simulink model "Circuit_Diagram"  (R2022a)
settings: Solver=VariableStepAuto  StartTime=0.0  StopTime=10.0  RelTol=1e-3
libraries: fl_lib x27, ee_lib x9
settings Model: Creator=Tony  LastModifiedBy=Tony

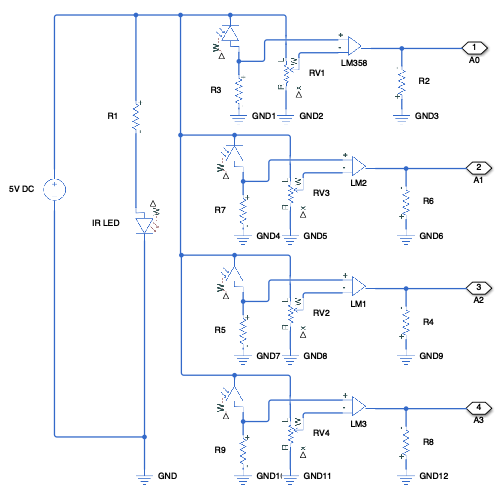
[thumbnail: Simulink's stored preview of the top-level diagram]
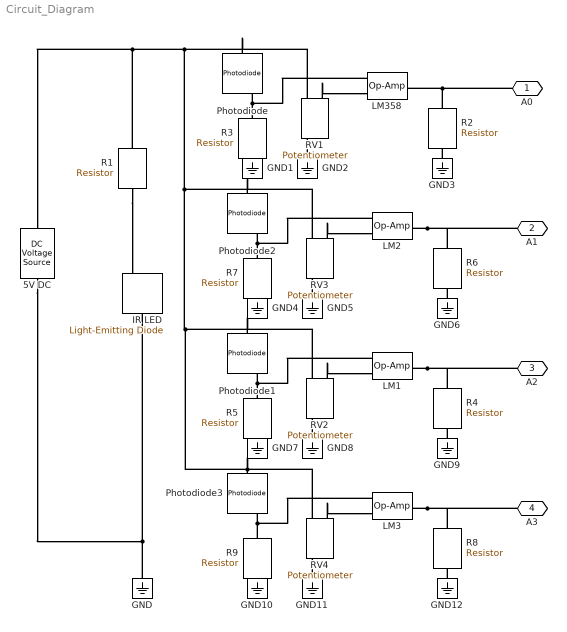
== system Circuit_Diagram ==
  5V DC : fl_lib/Electrical/Electrical Sources/DC Voltage Source  v0=5 V
      settings: SourceProductBaseCode=PW,SS,VE
  GND{,1..12} (13 alike) : fl_lib/Electrical/Electrical Elements/Electrical Reference
      settings: SourceProductBaseCode=PW,SS,VE
  "IR LED " : ee_lib/Sensors & Transducers/Light-Emitting Diode  Gain=0.005 W/A  prmExp=1  I12=[.0017, .003] A  V12=[.9, 1.05] V  IS=5e-5 A  ec=10  RS=0.1 Ohm  Tmeas=25 degC  C_param=1  CJ=20 pF  CJ0=20 pF  VJ=1 V  Mgrad=0.5  Vvec=[.1, 10, 100] V  Cvec=[15, 10, 2] pF  FC=0.5  T_param=1  IS_T2=1.8e-4 A  I1_T2=0.0034 A  V1_T2=1.05 V  Tmeas2=125 degC  EG_param=1  EG=1.11 eV  XTI_param=1  XTI=3  Tdevice=25 degC  i_capacitor_specify=off  i_capacitor_priority=High  i_capacitor=0 A  i_capacitor_nominal_specify=off  i_capacitor_nominal_unit=A  i_capacitor_nominal_value=1  v_capacitor_specify=off  v_capacitor_priority=None  v_capacitor=0 V  v_capacitor_nominal_specify=off  v_capacitor_nominal_unit=V  v_capacitor_nominal_value=1  thermal_network_parameterization=ee.enum.thermalNetworkTopology.junctionCase  Rth=[0, 10] K/W  Rth_Cauer=[1, 3, 10] K/W  Rth_Foster=[4, 6] K/W  thermal_mass_parameterization=ee.enum.thermalNetwork.timeconstant  thermal_mass=[0, 1] J/K  thermal_mass_Cauer=[1.5, 2, 3] J/K  thermal_mass_Foster=[1.5, 3] J/K  thermal_time_constant=[0, 10] s  thermal_time_constant_Cauer=[1, 3, 10] s  thermal_time_constant_Foster=[6, 18] s  thermal_mass_initial_temperatures=[25, 25] degC  thermal_mass_initial_temperatures_Cauer=[25, 25, 25] degC  steadyState_Foster=simscape.enum.onoff.on  Tvec_initial_Foster=[25, 25, 25, 25] degC
      settings: SourceProductBaseCode=PS  InternalSimscapePortConfiguration="{\"Bottom\":[],\"Left\":[{\"id\":\"W\",\"label\":\"W\",\"type\":\"output\"},{\"id\":\"p\",\"label\":\"\",\"type\":\"foundation.electrical.electrical\"}],\"Right\":[{\"id\":\"n\",\"label\":\"\",\"type\":\"foundation.electrical.electrical\"}],\"Top\":[]}"
  LM{1..3,358} (4 alike) : fl_lib/Electrical/Electrical Elements/Op-Amp  outI_specify=off  outI_priority=None  outI=0 A  outI_nominal_specify=off  outI_nominal_unit=A  outI_nominal_value=1
      settings: SourceProductBaseCode=PW,SS,VE
  Photodiode{,1..3} (4 alike) : ee_lib/Sensors & Transducers/Photodiode  prmFlux=1  Imeas=25 uA  FluxD=5 W/m^2  G=5e-6 A*m^2/W  prmExp=1  I2=0.1 A  V2=1.3 V  IS=5e-9 A  ec=3  RS=0.1 Ohm  Tmeas=25 degC  C_param=1  CJ=60 pF  CJ0=60 pF  VJ=1 V  Mgrad=0.5  Vvec=[.1, 10, 100] V  Cvec=[45, 3, 6] pF  FC=0.5  T_param=1  IS_T2=2.5e-7 A  I1_T2=0.07 A  V1_T2=1.3 V  Tmeas2=125 degC  EG_param=1  EG=1.11 eV  XTI_param=1  XTI=3  Tdevice=25 degC  i_capacitor_specify=off  i_capacitor_priority=High  i_capacitor=0 A  i_capacitor_nominal_specify=off  i_capacitor_nominal_unit=A  i_capacitor_nominal_value=1  v_capacitor_specify=off  v_capacitor_priority=None  v_capacitor=0 V  v_capacitor_nominal_specify=off  v_capacitor_nominal_unit=V  v_capacitor_nominal_value=1  thermal_network_parameterization=ee.enum.thermalNetworkTopology.junctionCase  Rth=[0, 10] K/W  Rth_Cauer=[1, 3, 10] K/W  Rth_Foster=[4, 6] K/W  thermal_mass_parameterization=ee.enum.thermalNetwork.timeconstant  thermal_mass=[0, 1] J/K  thermal_mass_Cauer=[1.5, 2, 3] J/K  thermal_mass_Foster=[1.5, 3] J/K  thermal_time_constant=[0, 10] s  thermal_time_constant_Cauer=[1, 3, 10] s  thermal_time_constant_Foster=[6, 18] s  thermal_mass_initial_temperatures=[25, 25] degC  thermal_mass_initial_temperatures_Cauer=[25, 25, 25] degC  steadyState_Foster=simscape.enum.onoff.on  Tvec_initial_Foster=[25, 25, 25, 25] degC
      settings: SourceProductBaseCode=PS  InternalSimscapePortConfiguration="{\"Bottom\":[],\"Left\":[{\"id\":\"W\",\"label\":\"W\",\"type\":\"input\"},{\"id\":\"p\",\"label\":\"\",\"type\":\"foundation.electrical.electrical\"}],\"Right\":[{\"id\":\"n\",\"label\":\"\",\"type\":\"foundation.electrical.electrical\"}],\"Top\":[]}"
  R{1,3,5,7,9} (5 alike) : fl_lib/Electrical/Electrical Elements/Resistor  R=100 Ohm  i_specify=off  i_priority=None  i=0 A  i_nominal_specify=off  i_nominal_unit=A  i_nominal_value=1  v_specify=off  v_priority=None  v=0 V  v_nominal_specify=off  v_nominal_unit=V  v_nominal_value=1
      settings: SourceProductBaseCode=PW,SS,VE
  R{2,4,6,8} (4 alike) : fl_lib/Electrical/Electrical Elements/Resistor  R=220 Ohm  i_specify=off  i_priority=None  i=0 A  i_nominal_specify=off  i_nominal_unit=A  i_nominal_value=1  v_specify=off  v_priority=None  v=0 V  v_nominal_specify=off  v_nominal_unit=V  v_nominal_value=1
      settings: SourceProductBaseCode=PW,SS,VE
  RV{1..4} (4 alike) : ee_lib/Passive/Potentiometer  R0=10000 Ohm  Rw=1 Ohm  xmin=0  xmax=1  Taper=ee.enum.linOrLog.lin  Rcenter=200 Ohm  Gradient=ee.enum.passive.potentiometer.gradient.higherR
      settings: SourceProductBaseCode=PS  InternalSimscapePortConfiguration="{\"Bottom\":[],\"Left\":[{\"id\":\"pinL\",\"label\":\"L\",\"type\":\"foundation.electrical.electrical\"},{\"id\":\"W\",\"label\":\"W\",\"type\":\"foundation.electrical.electrical\"}],\"Right\":[{\"id\":\"pinR\",\"label\":\"R\",\"type\":\"foundation.electrical.electrical\"},{\"id\":\"x\",\"label\":\"x\",\"type\":\"input\"}],\"Top\":[]}"
  A0 : PMIOPort  Side=Left
  A1 : PMIOPort  Port=2  Side=Left
  A2 : PMIOPort  Port=3  Side=Left
  A3 : PMIOPort  Port=4  Side=Left
  connections:
  R1/RConn1 -- "IR LED "/LConn2
  Photodiode3/RConn1 -- R1/LConn1 -- 5V DC/LConn1 -- RV1/LConn1 -- Photodiode/RConn1 -- RV3/LConn1 -- Photodiode2/RConn1 -- RV2/LConn1 -- Photodiode1/RConn1 -- RV4/LConn1
  GND/LConn1 -- 5V DC/RConn1 -- "IR LED "/RConn1
  R2/RConn1 -- A0/RConn1 -- LM358/RConn1
  RV1/LConn2 -- LM358/LConn2
  R3/LConn1 -- LM358/LConn1 -- Photodiode/LConn2
  GND1/LConn1 -- R3/RConn1
  GND2/LConn1 -- RV1/RConn1
  GND3/LConn1 -- R2/LConn1
  R7/LConn1 -- LM2/LConn1 -- Photodiode2/LConn2
  LM2/RConn1 -- A1/RConn1 -- R6/RConn1
  GND5/LConn1 -- RV3/RConn1
  GND6/LConn1 -- R6/LConn1
  RV3/LConn2 -- LM2/LConn2
  GND4/LConn1 -- R7/RConn1
  R5/LConn1 -- LM1/LConn1 -- Photodiode1/LConn2
  LM1/RConn1 -- A2/RConn1 -- R4/RConn1
  GND8/LConn1 -- RV2/RConn1
  GND9/LConn1 -- R4/LConn1
  RV2/LConn2 -- LM1/LConn2
  GND7/LConn1 -- R5/RConn1
  R9/LConn1 -- LM3/LConn1 -- Photodiode3/LConn2
  LM3/RConn1 -- A3/RConn1 -- R8/RConn1
  GND11/LConn1 -- RV4/RConn1
  GND12/LConn1 -- R8/LConn1
  RV4/LConn2 -- LM3/LConn2
  GND10/LConn1 -- R9/RConn1
